simulink model "task_1_sim"  (R2023a)
settings: Solver=VariableStepAuto  StartTime=0.0  StopTime=4  RelTol=1e-6
undefined symbols (not defined in the file): A, B, K2, x_0
settings Model: Creator=user  LastModifiedBy=user

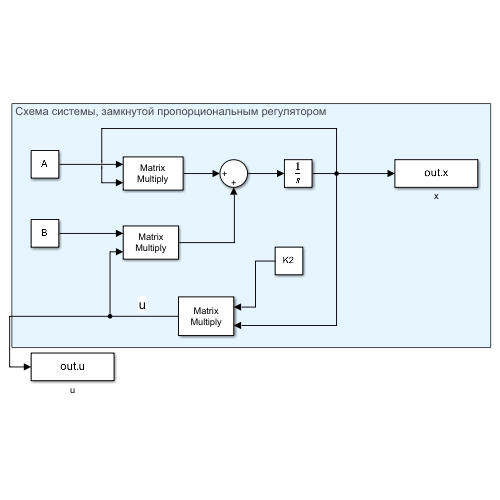
[thumbnail: Simulink's stored preview of the top-level diagram]
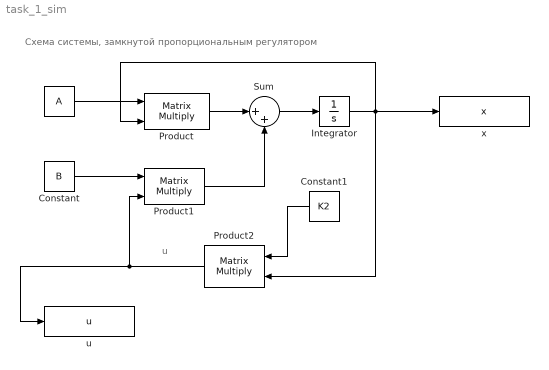
== system task_1_sim ==
  note: Схема системы, замкнутой пропорциональным регулятором
  note: u
  " " : Constant  Value=A
  Constant : Constant  Value=B  VectorParams1D=off
  Constant1 : Constant  Value=K2  VectorParams1D=off
  Integrator : Integrator  InitialCondition=x_0
  Product : Product  Multiplication=Matrix(*)
  Product1 : Product  Multiplication=Matrix(*)
  Product2 : Product  Multiplication=Matrix(*)
  Sum : Sum  Inputs=|++
  u : ToWorkspace  VariableName=u  SaveFormat=Timeseries  SampleTime=-1
  x : ToWorkspace  VariableName=x  SaveFormat=Timeseries  SampleTime=-1
  wires:
  " "/1 -> Product/1
  Constant/1 -> Product1/1
  Product/1 -> Sum/1
  Product1/1 -> Sum/2
  Sum/1 -> Integrator/1
  Integrator/1 -> Product2/2, Product/2, x/1
  Constant1/1 -> Product2/1
  Product2/1 -> Product1/2, u/1
